simulink model "PositionControl"  (R2019b)
settings: Solver=ode3  StartTime=0.0  StopTime=100.0  FixedStep=Ts  RelTol=1e-3
model workspace (MAT data in the model file):
  th_0 = 0
  x_0 = 0
  y_0 = 0
undefined symbols (not defined in the file): DiscIntNeverNeededParam, refx, refy
libraries: simulink x1
settings Model: Creator=pizarro  LastModifiedBy=Pablo
settings DataIOCC: SaveFormat=StructureWithTime  ReturnWorkspaceOutputs=off
settings SFSimCC: CustomCodeUndefinedFunction=UseInterfaceOnly

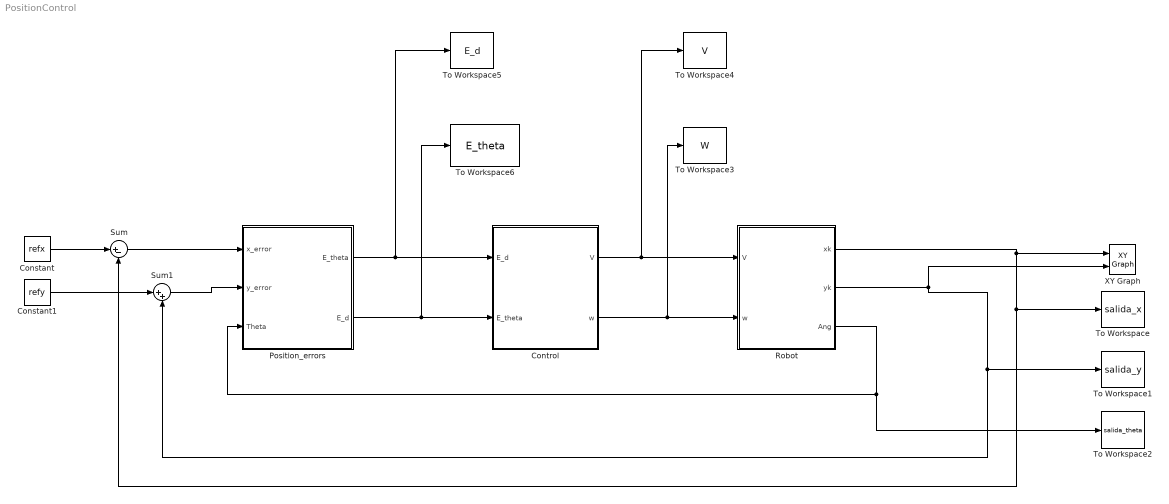
== system PositionControl ==
  Constant : Constant  Value=refx
  Constant1 : Constant  Value=refy
  Control : Subsystem
  Position_errors : Subsystem
  "Robot " : Subsystem
  Sum : Sum  Inputs=|+-
  Sum1 : Sum  Inputs=|++
  To Workspace : ToWorkspace  VariableName=salida_x  SaveFormat=Structure With Time  SampleTime=-1
      settings: Save2DSignal=2-D array (concatenate along first dimension)
  To Workspace1 : ToWorkspace  VariableName=salida_y  SaveFormat=Structure With Time  SampleTime=-1
      settings: Save2DSignal=2-D array (concatenate along first dimension)
  To Workspace2 : ToWorkspace  VariableName=salida_theta  SaveFormat=Structure With Time  SampleTime=-1
      settings: Save2DSignal=2-D array (concatenate along first dimension)
  To Workspace3 : ToWorkspace  VariableName=W  SaveFormat=Structure With Time  SampleTime=-1
      settings: Save2DSignal=2-D array (concatenate along first dimension)
  To Workspace4 : ToWorkspace  VariableName=V  SaveFormat=Structure With Time  SampleTime=-1
      settings: Save2DSignal=2-D array (concatenate along first dimension)
  To Workspace5 : ToWorkspace  VariableName=E_d  SaveFormat=Structure With Time  SampleTime=-1
      settings: Save2DSignal=2-D array (concatenate along first dimension)
  To Workspace6 : ToWorkspace  VariableName=E_theta  SaveFormat=Structure With Time  SampleTime=-1
      settings: Save2DSignal=2-D array (concatenate along first dimension)
  XY Graph : simulink/Sinks/XY Graph  xmin=-5  xmax=5  ymin=-5  ymax=5  st=-1
  wires:
  Position_errors/2(E_d) -> Control/2(E_theta), To Workspace6/1
  Position_errors/1(E_theta) -> Control/1(E_d), To Workspace5/1
  Control/2(w) -> To Workspace3/1, "Robot "/2("w ")
  Control/1(V) -> To Workspace4/1, "Robot "/1(V)
  "Robot "/3(Ang) -> To Workspace2/1, Position_errors/3(Theta)
  Constant/1 -> Sum/1
  Sum/1 -> Position_errors/1("x_error ")
  Sum1/1 -> Position_errors/2("y_error ")
  Constant1/1 -> Sum1/1
  "Robot "/1(xk) -> XY Graph/1, Sum/2, To Workspace/1
  "Robot "/2(yk) -> XY Graph/2, Sum1/2, To Workspace1/1

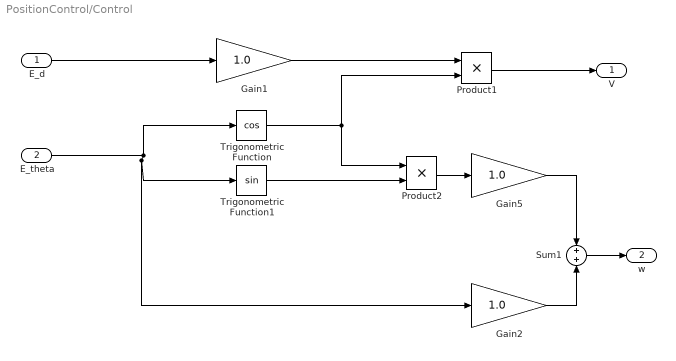
== system PositionControl/Control ==
  E_d : Inport
  E_theta : Inport  Port=2
  Gain1 : Gain  Gain=1.0
  Gain2 : Gain  Gain=1.0
  Gain5 : Gain  Gain=1.0
  Product1 : Product
  Product2 : Product
  Sum1 : Sum
  Trigonometric Function : Trigonometry  Operator=cos
  Trigonometric Function1 : Trigonometry
  V : Outport  VectorParamsAs1DForOutWhenUnconnected=off
  w : Outport  Port=2  VectorParamsAs1DForOutWhenUnconnected=off
  wires:
  E_theta/1 -> Trigonometric Function/1, Trigonometric Function1/1, Gain2/1
  E_d/1 -> Gain1/1
  Trigonometric Function/1 -> Product1/2, Product2/1
  Product1/1 -> V/1
  Trigonometric Function1/1 -> Product2/2
  Product2/1 -> Gain5/1
  Gain1/1 -> Product1/1
  Gain5/1 -> Sum1/1
  Gain2/1 -> Sum1/2
  Sum1/1 -> w/1

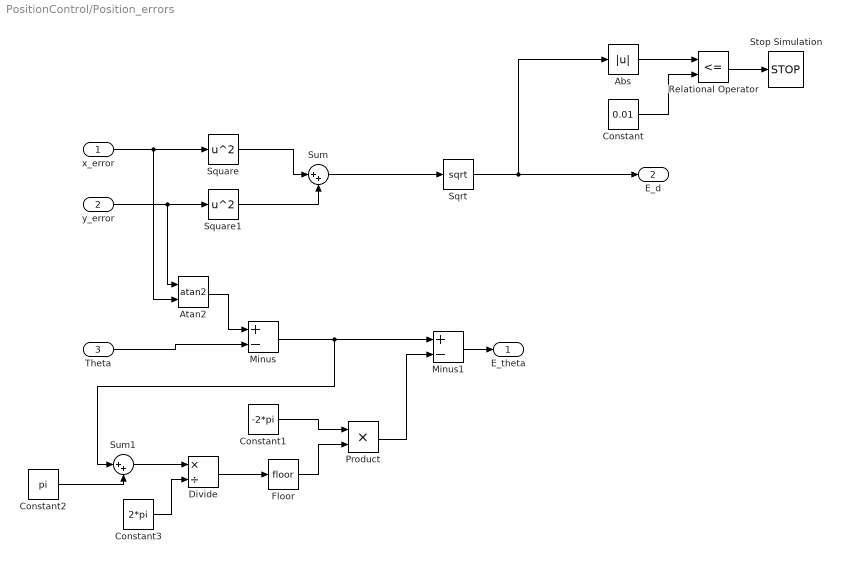
== system PositionControl/Position_errors ==
  "x_error " : Inport
  "y_error " : Inport  Port=2
  Theta : Inport  Port=3
  Abs : Abs
  Atan2 : Trigonometry  Operator=atan2
  Constant : Constant  Value=0.01
  Constant1 : Constant  Value=-2*pi
  Constant2 : Constant  Value=pi
  Constant3 : Constant  Value=2*pi
  Divide : Product  Inputs=*/
  Floor : Rounding
  Minus : Sum  Inputs=+-
  Minus1 : Sum  Inputs=+-
  Product : Product
  Relational Operator : RelationalOperator  Operator=<=  OutDataTypeStr=boolean  RndMeth=Simplest
  Sqrt : Sqrt  SaturateOnIntegerOverflow=on
  Square : Math  Operator=square  SaturateOnIntegerOverflow=on
  Square1 : Math  Operator=square  SaturateOnIntegerOverflow=on
  Stop Simulation : Stop
  Sum : Sum  Inputs=|++
  Sum1 : Sum  Inputs=|++
  E_theta : Outport
  E_d : Outport  Port=2
  wires:
  "x_error "/1 -> Atan2/2, Square/1
  Abs/1 -> Relational Operator/1
  Constant2/1 -> Sum1/2
  Constant/1 -> Relational Operator/2
  Constant1/1 -> Product/1
  "y_error "/1 -> Atan2/1, Square1/1
  Minus/1 -> Minus1/1, Sum1/1
  Theta/1 -> Minus/2
  Divide/1 -> Floor/1
  Sum/1 -> Sqrt/1
  Minus1/1 -> E_theta/1
  Sqrt/1 -> E_d/1, Abs/1
  Product/1 -> Minus1/2
  Constant3/1 -> Divide/2
  Floor/1 -> Product/2
  Square/1 -> Sum/1
  Square1/1 -> Sum/2
  Relational Operator/1 -> Stop Simulation/1
  Atan2/1 -> Minus/1
  Sum1/1 -> Divide/1

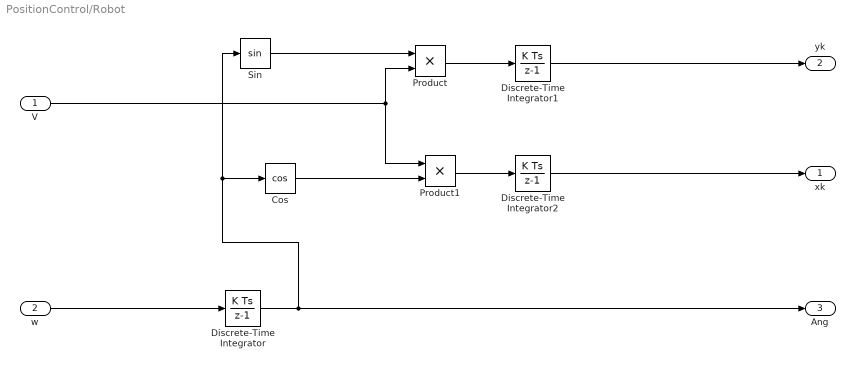
== system PositionControl/Robot  ==
  V : Inport
  "w " : Inport  Port=2
  Cos : Trigonometry  Operator=cos
  Discrete-Time Integrator : DiscreteIntegrator  SampleTime=-1  ICPrevOutput=DiscIntNeverNeededParam  ICPrevScaledInput=DiscIntNeverNeededParam
  Discrete-Time Integrator1 : DiscreteIntegrator  SampleTime=-1  ICPrevOutput=DiscIntNeverNeededParam  ICPrevScaledInput=DiscIntNeverNeededParam
  Discrete-Time Integrator2 : DiscreteIntegrator  SampleTime=-1  ICPrevOutput=DiscIntNeverNeededParam  ICPrevScaledInput=DiscIntNeverNeededParam
  Product : Product
  Product1 : Product
  Sin : Trigonometry
  xk : Outport  VectorParamsAs1DForOutWhenUnconnected=off
  yk : Outport  Port=2  VectorParamsAs1DForOutWhenUnconnected=off
  Ang : Outport  Port=3  VectorParamsAs1DForOutWhenUnconnected=off
  wires:
  Sin/1 -> Product/1
  Cos/1 -> Product1/2
  V/1 -> Product1/1, Product/2
  Product/1 -> Discrete-Time Integrator1/1
  Discrete-Time Integrator2/1 -> xk/1
  Discrete-Time Integrator1/1 -> yk/1
  Product1/1 -> Discrete-Time Integrator2/1
  "w "/1 -> Discrete-Time Integrator/1
  Discrete-Time Integrator/1 -> Ang/1, Cos/1, Sin/1
